simulink library "halin"  (R2021b)
settings: Solver=VariableStepAuto  StartTime=0.0  StopTime=10.0  RelTol=1e-3
undefined symbols (not defined in the file): KHAL_CAN1ABM1E2E_flg, KHAL_CAN1EPB1E2E_flg, KHAL_CAN1EPS1E2E_flg, KHAL_CAN1ESC1E2E_flg, KHAL_CAN1ESC5E2E_flg, KHAL_CAN3BMS1E2E_flg, KHAL_CAN3BMS6E2E_flg, KHAL_CAN3CCU1E2E_flg, KHAL_CAN3CCU2E2E_flg, KHAL_CAN3MCUNF1E2E_flg, KHAL_CAN3MCUNR1E2E_flg, KHAL_CAN3Shifter1E2E_flg, KHAL_CAN3Shifter2E2E_flg, KHAL_CAN6FCM2E2E_flg, KHAL_CAN6FCM4E2E_flg, TRUE
libraries: simulink x645, FVT_lib x212, hcu_lib x59
(part 4 of 23)

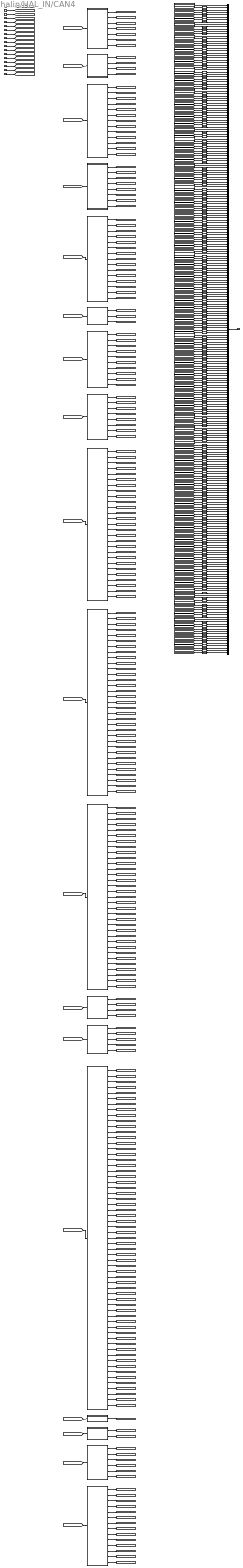
== system halin/HAL_IN/CAN4 ==
  DT_CAN4_SG_BodyZone_DR1 : Inport
  DT_CAN4_SG_BodyZone_DR2 : Inport  Port=2
  DT_CAN4_SG_BodyZone_PS1 : Inport  Port=3
  DT_CAN4_SG_BodyZone_PS2 : Inport  Port=4
  DT_CAN4_SG_DKC1 : Inport  Port=5
  DT_CAN4_SG_DKC2 : Inport  Port=6
  DT_CAN4_SG_PTG1 : Inport  Port=7
  DT_CAN4_SG_ZONE_DR1 : Inport  Port=8
  DT_CAN4_SG_ZONE_DR_VCU : Inport  Port=9
  DT_CAN4_SG_ZONE_FR1 : Inport  Port=10
  DT_CAN4_SG_ZONE_FR_VCU : Inport  Port=11
  DT_CAN4_SG_zGW_APTC1 : Inport  Port=12
  DT_CAN4_SG_zGW_CANFr1 : Inport  Port=13
  DT_CAN4_SG_zGW_LINDr1 : Inport  Port=14
  DT_CAN4_SG_zGW_LINDr2 : Inport  Port=15
  DT_CAN4_SG_zGW_LINFr1 : Inport  Port=16
  DT_CAN4_SG_zGW_LINFr2 : Inport  Port=17
  DT_CAN4_SG_zGW_SEAT1 : Inport  Port=18
  BodyZone_DR1 : Subsystem
  BodyZone_DR2 : Subsystem
  BodyZone_PS1 : Subsystem
  BodyZone_PS2 : Subsystem
  DKC1 : Subsystem
  DKC2 : Subsystem
  PTG1 : Subsystem
  UnitConverter{,1..2,9..11,16,19,26..27,44,46,51..52,55,60..62,64,66..67,69..72,95..97,99..100,102..119,121..123,138,170,173,177..179,182..183,186..187,190..191,194..195,197..231,240..242,248} (104 alike) : DataTypeConversion  OutDataTypeStr=boolean
  UnitConverter{7..8,21,24..25,56,63,65,74,76,78,80,82,84,86,88,90,92,98,101,124..127,129,131,139,141,143,145,147,149,151,153,159,161..169,180,184,188,192} (48 alike) : DataTypeConversion  OutDataTypeStr=single
  UnitConverter{3..6,12..15,17..18,22..23,28..43,45,50,53..54,57..59,68,75,77,79,81,83,85,87,89,91,93..94,120,128,130,132..137,140,142,144,146,148,150,152,154..158,160,171..172,174..176,181,185,189,193,196,232..239,244,246..247,250,252..253} (93 alike) : DataTypeConversion  OutDataTypeStr=uint8
  UnitConverter{20,73,243,245,249,251} (6 alike) : DataTypeConversion  OutDataTypeStr=uint16
  UnitConverter47 : DataTypeConversion  OutDataTypeStr=uint64
  UnitConverter48 : DataTypeConversion  OutDataTypeStr=uint64
  UnitConverter49 : DataTypeConversion  OutDataTypeStr=uint64
  VHAL_CANMsgInvalidBodyZoneDR1_flg : Subsystem  AncestorBlock=FVT_lib/hal/MsgTimeoutJudge_CAN_AUTOSAR
      mask help: MeasumentTrigerEvent
      mask Display: fprintf('MsgTimeoutJudge_CAN\nAUTOSAR');
  VHAL_CANMsgInvalidBodyZoneDR2_flg : Subsystem  AncestorBlock=FVT_lib/hal/MsgTimeoutJudge_CAN_AUTOSAR
      mask help: MeasumentTrigerEvent
      mask Display: fprintf('MsgTimeoutJudge_CAN\nAUTOSAR');
  VHAL_CANMsgInvalidBodyZonePS1_flg : Subsystem  AncestorBlock=FVT_lib/hal/MsgTimeoutJudge_CAN_AUTOSAR
      mask help: MeasumentTrigerEvent
      mask Display: fprintf('MsgTimeoutJudge_CAN\nAUTOSAR');
  VHAL_CANMsgInvalidBodyZonePS2_flg : Subsystem  AncestorBlock=FVT_lib/hal/MsgTimeoutJudge_CAN_AUTOSAR
      mask help: MeasumentTrigerEvent
      mask Display: fprintf('MsgTimeoutJudge_CAN\nAUTOSAR');
  VHAL_CANMsgInvalidDKC1_flg : Subsystem  AncestorBlock=FVT_lib/hal/MsgTimeoutJudge_CAN_AUTOSAR
      mask help: MeasumentTrigerEvent
      mask Display: fprintf('MsgTimeoutJudge_CAN\nAUTOSAR');
  VHAL_CANMsgInvalidDKC2_flg : Subsystem  AncestorBlock=FVT_lib/hal/MsgTimeoutJudge_CAN_AUTOSAR
      mask help: MeasumentTrigerEvent
      mask Display: fprintf('MsgTimeoutJudge_CAN\nAUTOSAR');
  VHAL_CANMsgInvalidPTG1_flg : Subsystem  AncestorBlock=FVT_lib/hal/MsgTimeoutJudge_CAN_AUTOSAR
      mask help: MeasumentTrigerEvent
      mask Display: fprintf('MsgTimeoutJudge_CAN\nAUTOSAR');
  VHAL_CANMsgInvalidZONEDR1_flg : Subsystem  AncestorBlock=FVT_lib/hal/MsgTimeoutJudge_CAN_AUTOSAR
      mask help: MeasumentTrigerEvent
      mask Display: fprintf('MsgTimeoutJudge_CAN\nAUTOSAR');
  VHAL_CANMsgInvalidZONEDRVCU_flg : Subsystem  AncestorBlock=FVT_lib/hal/MsgTimeoutJudge_CAN_AUTOSAR
      mask help: MeasumentTrigerEvent
      mask Display: fprintf('MsgTimeoutJudge_CAN\nAUTOSAR');
  VHAL_CANMsgInvalidZONEFR1_flg : Subsystem  AncestorBlock=FVT_lib/hal/MsgTimeoutJudge_CAN_AUTOSAR
      mask help: MeasumentTrigerEvent
      mask Display: fprintf('MsgTimeoutJudge_CAN\nAUTOSAR');
  VHAL_CANMsgInvalidZONEFRVCU_flg : Subsystem  AncestorBlock=FVT_lib/hal/MsgTimeoutJudge_CAN_AUTOSAR
      mask help: MeasumentTrigerEvent
      mask Display: fprintf('MsgTimeoutJudge_CAN\nAUTOSAR');
  VHAL_CANMsgInvalidzGWAPTC1_flg : Subsystem  AncestorBlock=FVT_lib/hal/MsgTimeoutJudge_CAN_AUTOSAR
      mask help: MeasumentTrigerEvent
      mask Display: fprintf('MsgTimeoutJudge_CAN\nAUTOSAR');
  VHAL_CANMsgInvalidzGWCANFr1_flg : Subsystem  AncestorBlock=FVT_lib/hal/MsgTimeoutJudge_CAN_AUTOSAR
      mask help: MeasumentTrigerEvent
      mask Display: fprintf('MsgTimeoutJudge_CAN\nAUTOSAR');
  VHAL_CANMsgInvalidzGWLINDr1_flg : Subsystem  AncestorBlock=FVT_lib/hal/MsgTimeoutJudge_CAN_AUTOSAR
      mask help: MeasumentTrigerEvent
      mask Display: fprintf('MsgTimeoutJudge_CAN\nAUTOSAR');
  VHAL_CANMsgInvalidzGWLINDr2_flg : Subsystem  AncestorBlock=FVT_lib/hal/MsgTimeoutJudge_CAN_AUTOSAR
      mask help: MeasumentTrigerEvent
      mask Display: fprintf('MsgTimeoutJudge_CAN\nAUTOSAR');
  VHAL_CANMsgInvalidzGWLINFr1_flg : Subsystem  AncestorBlock=FVT_lib/hal/MsgTimeoutJudge_CAN_AUTOSAR
      mask help: MeasumentTrigerEvent
      mask Display: fprintf('MsgTimeoutJudge_CAN\nAUTOSAR');
  VHAL_CANMsgInvalidzGWLINFr2_flg : Subsystem  AncestorBlock=FVT_lib/hal/MsgTimeoutJudge_CAN_AUTOSAR
      mask help: MeasumentTrigerEvent
      mask Display: fprintf('MsgTimeoutJudge_CAN\nAUTOSAR');
  VHAL_CANMsgInvalidzGWSEAT1_flg : Subsystem  AncestorBlock=FVT_lib/hal/MsgTimeoutJudge_CAN_AUTOSAR
      mask help: MeasumentTrigerEvent
      mask Display: fprintf('MsgTimeoutJudge_CAN\nAUTOSAR');
  ZONE_DR1 : Subsystem
  ZONE_DR_VCU : Subsystem
  ZONE_FR1 : Subsystem
  ZONE_FR_VCU : Subsystem
  bus_creator : BusCreator  Inputs=272
  zGW_APTC1 : Subsystem
  zGW_CANFr1 : Subsystem
  zGW_LINDr1 : Subsystem
  zGW_LINDr2 : Subsystem
  zGW_LINFr1 : Subsystem
  zGW_LINFr2 : Subsystem
  zGW_SEAT1 : Subsystem
  HAL_CAN4_outputs : Outport
  wires:
  DT_CAN4_SG_BodyZone_DR1/1 -> [DT_CAN4_SG_BodyZone_DR1]
  DT_CAN4_SG_BodyZone_DR2/1 -> [DT_CAN4_SG_BodyZone_DR2]
  DT_CAN4_SG_BodyZone_PS1/1 -> [DT_CAN4_SG_BodyZone_PS1]
  DT_CAN4_SG_BodyZone_PS2/1 -> [DT_CAN4_SG_BodyZone_PS2]
  DT_CAN4_SG_DKC1/1 -> [DT_CAN4_SG_DKC1]
  DT_CAN4_SG_DKC2/1 -> [DT_CAN4_SG_DKC2]
  DT_CAN4_SG_PTG1/1 -> [DT_CAN4_SG_PTG1]
  DT_CAN4_SG_ZONE_DR1/1 -> [DT_CAN4_SG_ZONE_DR1]
  DT_CAN4_SG_ZONE_DR_VCU/1 -> [DT_CAN4_SG_ZONE_DR_VCU]
  DT_CAN4_SG_ZONE_FR1/1 -> [DT_CAN4_SG_ZONE_FR1]
  DT_CAN4_SG_ZONE_FR_VCU/1 -> [DT_CAN4_SG_ZONE_FR_VCU]
  DT_CAN4_SG_zGW_APTC1/1 -> [DT_CAN4_SG_zGW_APTC1]
  DT_CAN4_SG_zGW_CANFr1/1 -> [DT_CAN4_SG_zGW_CANFr1]
  DT_CAN4_SG_zGW_LINDr1/1 -> [DT_CAN4_SG_zGW_LINDr1]
  DT_CAN4_SG_zGW_LINDr2/1 -> [DT_CAN4_SG_zGW_LINDr2]
  DT_CAN4_SG_zGW_LINFr1/1 -> [DT_CAN4_SG_zGW_LINFr1]
  DT_CAN4_SG_zGW_LINFr2/1 -> [DT_CAN4_SG_zGW_LINFr2]
  DT_CAN4_SG_zGW_SEAT1/1 -> [DT_CAN4_SG_zGW_SEAT1]
  [DT_CAN4_SG_BodyZone_DR1] -> BodyZone_DR1/1(DT_CAN4_SG_BodyZone_DR1)
  [DT_CAN4_SG_BodyZone_DR2] -> BodyZone_DR2/1(DT_CAN4_SG_BodyZone_DR2)
  [DT_CAN4_SG_BodyZone_PS1] -> BodyZone_PS1/1(DT_CAN4_SG_BodyZone_PS1)
  [DT_CAN4_SG_BodyZone_PS2] -> BodyZone_PS2/1(DT_CAN4_SG_BodyZone_PS2)
  [DT_CAN4_SG_DKC1] -> DKC1/1(DT_CAN4_SG_DKC1)
  [DT_CAN4_SG_DKC2] -> DKC2/1(DT_CAN4_SG_DKC2)
  [DT_CAN4_SG_PTG1] -> PTG1/1(DT_CAN4_SG_PTG1)
  [DT_CAN4_SG_ZONE_DR1] -> ZONE_DR1/1(DT_CAN4_SG_ZONE_DR1)
  [DT_CAN4_SG_ZONE_DR_VCU] -> ZONE_DR_VCU/1(DT_CAN4_SG_ZONE_DR_VCU)
  [DT_CAN4_SG_ZONE_FR1] -> ZONE_FR1/1(DT_CAN4_SG_ZONE_FR1)
  [DT_CAN4_SG_ZONE_FR_VCU] -> ZONE_FR_VCU/1(DT_CAN4_SG_ZONE_FR_VCU)
  [DT_CAN4_SG_zGW_APTC1] -> zGW_APTC1/1(DT_CAN4_SG_zGW_APTC1)
  [DT_CAN4_SG_zGW_CANFr1] -> zGW_CANFr1/1(DT_CAN4_SG_zGW_CANFr1)
  [DT_CAN4_SG_zGW_LINDr1] -> zGW_LINDr1/1(DT_CAN4_SG_zGW_LINDr1)
  [DT_CAN4_SG_zGW_LINDr2] -> zGW_LINDr2/1(DT_CAN4_SG_zGW_LINDr2)
  [DT_CAN4_SG_zGW_LINFr1] -> zGW_LINFr1/1(DT_CAN4_SG_zGW_LINFr1)
  [DT_CAN4_SG_zGW_LINFr2] -> zGW_LINFr2/1(DT_CAN4_SG_zGW_LINFr2)
  [DT_CAN4_SG_zGW_SEAT1] -> zGW_SEAT1/1(DT_CAN4_SG_zGW_SEAT1)
  bus_creator/1 -> HAL_CAN4_outputs/1
  VHAL_CANMsgInvalidBodyZoneDR1_flg/1(Out) -> bus_creator/1
  BodyZone_DR1/1(VHAL_BDDSEATAntiSta_flg) -> [VHAL_BDDSEATAntiSta_flg]
  UnitConverter/1 -> bus_creator/2  "VHAL_BDDSEATAntiSta_flg"
  [VHAL_BDDSEATAntiSta_flg] -> UnitConverter/1
  BodyZone_DR1/2(VHAL_BDDSEATEntryFunSta_flg) -> [VHAL_BDDSEATEntryFunSta_flg]
  UnitConverter1/1 -> bus_creator/3  "VHAL_BDDSEATEntryFunSta_flg"
  [VHAL_BDDSEATEntryFunSta_flg] -> UnitConverter1/1
  BodyZone_DR1/3(VHAL_BDDSEATErrorSta_flg) -> [VHAL_BDDSEATErrorSta_flg]
  UnitConverter2/1 -> bus_creator/4  "VHAL_BDDSEATErrorSta_flg"
  [VHAL_BDDSEATErrorSta_flg] -> UnitConverter2/1
  BodyZone_DR1/4(VHAL_BDDSEATMemSetSta_enum) -> [VHAL_BDDSEATMemSetSta_enum]
  UnitConverter3/1 -> bus_creator/5  "VHAL_BDDSEATMemSetSta_enum"
  [VHAL_BDDSEATMemSetSta_enum] -> UnitConverter3/1
  BodyZone_DR1/5(VHAL_BDDSEATModeSta_enum) -> [VHAL_BDDSEATModeSta_enum]
  UnitConverter4/1 -> bus_creator/6  "VHAL_BDDSEATModeSta_enum"
  [VHAL_BDDSEATModeSta_enum] -> UnitConverter4/1
  BodyZone_DR1/6(VHAL_BDDSEATVentSta_enum) -> [VHAL_BDDSEATVentSta_enum]
  UnitConverter5/1 -> bus_creator/7  "VHAL_BDDSEATVentSta_enum"
  [VHAL_BDDSEATVentSta_enum] -> UnitConverter5/1
  BodyZone_DR1/7(VHAL_BDDSEATheaterSta_enum) -> [VHAL_BDDSEATheaterSta_enum]
  UnitConverter6/1 -> bus_creator/8  "VHAL_BDDSEATheaterSta_enum"
  [VHAL_BDDSEATheaterSta_enum] -> UnitConverter6/1
  VHAL_CANMsgInvalidBodyZoneDR2_flg/1(Out) -> bus_creator/9
  BodyZone_DR2/1(VHAL_BDAPMWinFOpenedSta_pct) -> [VHAL_BDAPMWinFOpenedSta_pct]
  UnitConverter7/1 -> bus_creator/10  "VHAL_BDAPMWinFOpenedSta_pct"
  [VHAL_BDAPMWinFOpenedSta_pct] -> UnitConverter7/1
  BodyZone_DR2/2(VHAL_BDAPMWinROpenedSta_pct) -> [VHAL_BDAPMWinROpenedSta_pct]
  UnitConverter8/1 -> bus_creator/11  "VHAL_BDAPMWinROpenedSta_pct"
  [VHAL_BDAPMWinROpenedSta_pct] -> UnitConverter8/1
  BodyZone_DR2/3(VHAL_BDDoorFHandleCloseSta_flg) -> [VHAL_BDDoorFHandleCloseSta_flg]
  UnitConverter9/1 -> bus_creator/12  "VHAL_BDDoorFHandleCloseSta_flg"
  [VHAL_BDDoorFHandleCloseSta_flg] -> UnitConverter9/1
  BodyZone_DR2/4(VHAL_BDDoorRHandleCloseSta_flg) -> [VHAL_BDDoorRHandleCloseSta_flg]
  UnitConverter10/1 -> bus_creator/13  "VHAL_BDDoorRHandleCloseSta_flg"
  [VHAL_BDDoorRHandleCloseSta_flg] -> UnitConverter10/1
  VHAL_CANMsgInvalidBodyZonePS1_flg/1(Out) -> bus_creator/14
  BodyZone_PS1/1(VHAL_BPPSEATErrorSta_flg) -> [VHAL_BPPSEATErrorSta_flg]
  UnitConverter11/1 -> bus_creator/15  "VHAL_BPPSEATErrorSta_flg"
  [VHAL_BPPSEATErrorSta_flg] -> UnitConverter11/1
  BodyZone_PS1/2(VHAL_BPPSEATModeSta_enum) -> [VHAL_BPPSEATModeSta_enum]
  UnitConverter12/1 -> bus_creator/16  "VHAL_BPPSEATModeSta_enum"
  [VHAL_BPPSEATModeSta_enum] -> UnitConverter12/1
  BodyZone_PS1/3(VHAL_BPPSEATVentSta_enum) -> [VHAL_BPPSEATVentSta_enum]
  UnitConverter13/1 -> bus_creator/17  "VHAL_BPPSEATVentSta_enum"
  [VHAL_BPPSEATVentSta_enum] -> UnitConverter13/1
  BodyZone_PS1/4(VHAL_BPPSEATheaterSta_enum) -> [VHAL_BPPSEATheaterSta_enum]
  UnitConverter14/1 -> bus_creator/18  "VHAL_BPPSEATheaterSta_enum"
  [VHAL_BPPSEATheaterSta_enum] -> UnitConverter14/1
  BodyZone_PS1/5(VHAL_BPPTGActiveSta_enum) -> [VHAL_BPPTGActiveSta_enum]
  UnitConverter15/1 -> bus_creator/19  "VHAL_BPPTGActiveSta_enum"
  [VHAL_BPPTGActiveSta_enum] -> UnitConverter15/1
  BodyZone_PS1/6(VHAL_BPPTGExistSta_flg) -> [VHAL_BPPTGExistSta_flg]
  UnitConverter16/1 -> bus_creator/20  "VHAL_BPPTGExistSta_flg"
  [VHAL_BPPTGExistSta_flg] -> UnitConverter16/1
  BodyZone_PS1/7(VHAL_BPPTGInsideSW1Sta_enum) -> [VHAL_BPPTGInsideSW1Sta_enum]
  UnitConverter17/1 -> bus_creator/21  "VHAL_BPPTGInsideSW1Sta_enum"
  [VHAL_BPPTGInsideSW1Sta_enum] -> UnitConverter17/1
  BodyZone_PS1/8(VHAL_BPPTGInsideSW2Sta_enum) -> [VHAL_BPPTGInsideSW2Sta_enum]
  UnitConverter18/1 -> bus_creator/22  "VHAL_BPPTGInsideSW2Sta_enum"
  [VHAL_BPPTGInsideSW2Sta_enum] -> UnitConverter18/1
  BodyZone_PS1/9(VHAL_BPPTGIsSetHeightSta_flg) -> [VHAL_BPPTGIsSetHeightSta_flg]
  UnitConverter19/1 -> bus_creator/23  "VHAL_BPPTGIsSetHeightSta_flg"
  [VHAL_BPPTGIsSetHeightSta_flg] -> UnitConverter19/1
  BodyZone_PS1/10(VHAL_BPPTGLeftHallPosnSta_enum) -> [VHAL_BPPTGLeftHallPosnSta_enum]
  UnitConverter20/1 -> bus_creator/24  "VHAL_BPPTGLeftHallPosnSta_enum"
  [VHAL_BPPTGLeftHallPosnSta_enum] -> UnitConverter20/1
  BodyZone_PS1/11(VHAL_BPPTGOpenRatioSta_pct) -> [VHAL_BPPTGOpenRatioSta_pct]
  UnitConverter21/1 -> bus_creator/25  "VHAL_BPPTGOpenRatioSta_pct"
  [VHAL_BPPTGOpenRatioSta_pct] -> UnitConverter21/1
  BodyZone_PS1/12(VHAL_BPPTGRDILCmd_enum) -> [VHAL_BPPTGRDILCmd_enum]
  UnitConverter22/1 -> bus_creator/26  "VHAL_BPPTGRDILCmd_enum"
  [VHAL_BPPTGRDILCmd_enum] -> UnitConverter22/1
  BodyZone_PS1/13(VHAL_BPPTGSysSta_enum) -> [VHAL_BPPTGSysSta_enum]
  UnitConverter23/1 -> bus_creator/27  "VHAL_BPPTGSysSta_enum"
  [VHAL_BPPTGSysSta_enum] -> UnitConverter23/1
  VHAL_CANMsgInvalidBodyZonePS2_flg/1(Out) -> bus_creator/28
  BodyZone_PS2/1(VHAL_BPAPMWinFOpenedSta_pct) -> [VHAL_BPAPMWinFOpenedSta_pct]
  UnitConverter24/1 -> bus_creator/29  "VHAL_BPAPMWinFOpenedSta_pct"
  [VHAL_BPAPMWinFOpenedSta_pct] -> UnitConverter24/1
  BodyZone_PS2/2(VHAL_BPAPMWinROpenedSta_pct) -> [VHAL_BPAPMWinROpenedSta_pct]
  UnitConverter25/1 -> bus_creator/30  "VHAL_BPAPMWinROpenedSta_pct"
  [VHAL_BPAPMWinROpenedSta_pct] -> UnitConverter25/1
  BodyZone_PS2/3(VHAL_BPDoorFHandleCloseSta_flg) -> [VHAL_BPDoorFHandleCloseSta_flg]
  UnitConverter26/1 -> bus_creator/31  "VHAL_BPDoorFHandleCloseSta_flg"
  [VHAL_BPDoorFHandleCloseSta_flg] -> UnitConverter26/1
  BodyZone_PS2/4(VHAL_BPDoorRHandleCloseSta_flg) -> [VHAL_BPDoorRHandleCloseSta_flg]
  UnitConverter27/1 -> bus_creator/32  "VHAL_BPDoorRHandleCloseSta_flg"
  [VHAL_BPDoorRHandleCloseSta_flg] -> UnitConverter27/1
  BodyZone_PS2/5(VHAL_BPSEATLVentSta_enum) -> [VHAL_BPSEATLVentSta_enum]
  UnitConverter28/1 -> bus_creator/33  "VHAL_BPSEATLVentSta_enum"
  [VHAL_BPSEATLVentSta_enum] -> UnitConverter28/1
  BodyZone_PS2/6(VHAL_BPSEATMLVentSta_enum) -> [VHAL_BPSEATMLVentSta_enum]
  UnitConverter29/1 -> bus_creator/34  "VHAL_BPSEATMLVentSta_enum"
  [VHAL_BPSEATMLVentSta_enum] -> UnitConverter29/1
  BodyZone_PS2/7(VHAL_BPSEATMRVentSta_enum) -> [VHAL_BPSEATMRVentSta_enum]
  UnitConverter30/1 -> bus_creator/35  "VHAL_BPSEATMRVentSta_enum"
  [VHAL_BPSEATMRVentSta_enum] -> UnitConverter30/1
  BodyZone_PS2/8(VHAL_BPSEATRVentSta_enum) -> [VHAL_BPSEATRVentSta_enum]
  UnitConverter31/1 -> bus_creator/36  "VHAL_BPSEATRVentSta_enum"
  [VHAL_BPSEATRVentSta_enum] -> UnitConverter31/1
  VHAL_CANMsgInvalidDKC1_flg/1(Out) -> bus_creator/37
  DKC1/1(VHAL_DKCKeyNumSta_enum) -> [VHAL_DKCKeyNumSta_enum]
  UnitConverter32/1 -> bus_creator/38  "VHAL_DKCKeyNumSta_enum"
  [VHAL_DKCKeyNumSta_enum] -> UnitConverter32/1
  DKC1/2(VHAL_DKCKeyTypeSta_enum) -> [VHAL_DKCKeyTypeSta_enum]
  UnitConverter33/1 -> bus_creator/39  "VHAL_DKCKeyTypeSta_enum"
  [VHAL_DKCKeyTypeSta_enum] -> UnitConverter33/1
  DKC1/3(VHAL_DKCPDkeyAreaRAPSSta_enum) -> [VHAL_DKCPDkeyAreaRAPSSta_enum]
  UnitConverter34/1 -> bus_creator/40  "VHAL_DKCPDkeyAreaRAPSSta_enum"
  [VHAL_DKCPDkeyAreaRAPSSta_enum] -> UnitConverter34/1
  DKC1/4(VHAL_DKCParkingModeCmd_enum) -> [VHAL_DKCParkingModeCmd_enum]
  UnitConverter35/1 -> bus_creator/41  "VHAL_DKCParkingModeCmd_enum"
  [VHAL_DKCParkingModeCmd_enum] -> UnitConverter35/1
  DKC1/5(VHAL_DKCReVehData_enum) -> [VHAL_DKCReVehData_enum]
  UnitConverter36/1 -> bus_creator/42  "VHAL_DKCReVehData_enum"
  [VHAL_DKCReVehData_enum] -> UnitConverter36/1
  DKC1/6(VHAL_PCommandToBCM_enum) -> [VHAL_PCommandToBCM_enum]
  UnitConverter37/1 -> bus_creator/43  "VHAL_PCommandToBCM_enum"
  [VHAL_PCommandToBCM_enum] -> UnitConverter37/1
  DKC1/7(VHAL_PCommandToPTG_enum) -> [VHAL_PCommandToPTG_enum]
  UnitConverter38/1 -> bus_creator/44  "VHAL_PCommandToPTG_enum"
  [VHAL_PCommandToPTG_enum] -> UnitConverter38/1
  DKC1/8(VHAL_PDKeyAreaLockUnlock_enum) -> [VHAL_PDKeyAreaLockUnlock_enum]
  UnitConverter39/1 -> bus_creator/45  "VHAL_PDKeyAreaLockUnlock_enum"
  [VHAL_PDKeyAreaLockUnlock_enum] -> UnitConverter39/1
  DKC1/9(VHAL_PDKeyAreaPS_enum) -> [VHAL_PDKeyAreaPS_enum]
  UnitConverter40/1 -> bus_creator/46  "VHAL_PDKeyAreaPS_enum"
  [VHAL_PDKeyAreaPS_enum] -> UnitConverter40/1
  DKC1/10(VHAL_PDKeyAreaPTG_enum) -> [VHAL_PDKeyAreaPTG_enum]
  UnitConverter41/1 -> bus_creator/47  "VHAL_PDKeyAreaPTG_enum"
  [VHAL_PDKeyAreaPTG_enum] -> UnitConverter41/1
  DKC1/11(VHAL_PDKeyWelcome_enum) -> [VHAL_PDKeyWelcome_enum]
  UnitConverter42/1 -> bus_creator/48  "VHAL_PDKeyWelcome_enum"
  [VHAL_PDKeyWelcome_enum] -> UnitConverter42/1
  DKC1/12(VHAL_PDkeyShowIVI_enum) -> [VHAL_PDkeyShowIVI_enum]
  UnitConverter43/1 -> bus_creator/49  "VHAL_PDkeyShowIVI_enum"
  [VHAL_PDkeyShowIVI_enum] -> UnitConverter43/1
  DKC1/13(VHAL_PKeyMiss_flg) -> [VHAL_PKeyMiss_flg]
  UnitConverter44/1 -> bus_creator/50  "VHAL_PKeyMiss_flg"
  [VHAL_PKeyMiss_flg] -> UnitConverter44/1
  DKC1/14(VHAL_PKeyMode_enum) -> [VHAL_PKeyMode_enum]
  UnitConverter45/1 -> bus_creator/51  "VHAL_PKeyMode_enum"
  [VHAL_PKeyMode_enum] -> UnitConverter45/1
  DKC1/15(VHAL_PUIDLowPower_flg) -> [VHAL_PUIDLowPower_flg]
  UnitConverter46/1 -> bus_creator/52  "VHAL_PUIDLowPower_flg"
  [VHAL_PUIDLowPower_flg] -> UnitConverter46/1
  VHAL_CANMsgInvalidDKC2_flg/1(Out) -> bus_creator/53
  DKC2/1(VHAL_EncryptionDATA063_enum) -> [VHAL_EncryptionDATA063_enum]
  UnitConverter47/1 -> bus_creator/54  "VHAL_EncryptionDATA063_enum"
  [VHAL_EncryptionDATA063_enum] -> UnitConverter47/1
  DKC2/2(VHAL_EncryptionDATA64127_enum) -> [VHAL_EncryptionDATA64127_enum]
  UnitConverter48/1 -> bus_creator/55  "VHAL_EncryptionDATA64127_enum"
  [VHAL_EncryptionDATA64127_enum] -> UnitConverter48/1
  DKC2/3(VHAL_RandomNumberX_enum) -> [VHAL_RandomNumberX_enum]
  UnitConverter49/1 -> bus_creator/56  "VHAL_RandomNumberX_enum"
  [VHAL_RandomNumberX_enum] -> UnitConverter49/1
  VHAL_CANMsgInvalidPTG1_flg/1(Out) -> bus_creator/57
  PTG1/1(VHAL_PTGActiveSta_enum) -> [VHAL_PTGActiveSta_enum]
  UnitConverter50/1 -> bus_creator/58  "VHAL_PTGActiveSta_enum"
  [VHAL_PTGActiveSta_enum] -> UnitConverter50/1
  PTG1/2(VHAL_PTGAutoStaus_flg) -> [VHAL_PTGAutoStaus_flg]
  UnitConverter51/1 -> bus_creator/59  "VHAL_PTGAutoStaus_flg"
  [VHAL_PTGAutoStaus_flg] -> UnitConverter51/1
  PTG1/3(VHAL_PTGExist_flg) -> [VHAL_PTGExist_flg]
  UnitConverter52/1 -> bus_creator/60  "VHAL_PTGExist_flg"
  [VHAL_PTGExist_flg] -> UnitConverter52/1
  PTG1/4(VHAL_PTGHWVer_enum) -> [VHAL_PTGHWVer_enum]
  UnitConverter53/1 -> bus_creator/61  "VHAL_PTGHWVer_enum"
  [VHAL_PTGHWVer_enum] -> UnitConverter53/1
  PTG1/5(VHAL_PTGInnerSW2_enum) -> [VHAL_PTGInnerSW2_enum]
  UnitConverter54/1 -> bus_creator/62  "VHAL_PTGInnerSW2_enum"
  [VHAL_PTGInnerSW2_enum] -> UnitConverter54/1
  PTG1/6(VHAL_PTGIsSetHeight_flg) -> [VHAL_PTGIsSetHeight_flg]
  UnitConverter55/1 -> bus_creator/63  "VHAL_PTGIsSetHeight_flg"
  [VHAL_PTGIsSetHeight_flg] -> UnitConverter55/1
  PTG1/7(VHAL_PTGOpenRatio_pct) -> [VHAL_PTGOpenRatio_pct]
  UnitConverter56/1 -> bus_creator/64  "VHAL_PTGOpenRatio_pct"
  [VHAL_PTGOpenRatio_pct] -> UnitConverter56/1
  PTG1/8(VHAL_PTGRDILSta_enum) -> [VHAL_PTGRDILSta_enum]
  UnitConverter57/1 -> bus_creator/65  "VHAL_PTGRDILSta_enum"
  [VHAL_PTGRDILSta_enum] -> UnitConverter57/1
  PTG1/9(VHAL_PTGSWVer_enum) -> [VHAL_PTGSWVer_enum]
  UnitConverter58/1 -> bus_creator/66  "VHAL_PTGSWVer_enum"
  [VHAL_PTGSWVer_enum] -> UnitConverter58/1
  PTG1/10(VHAL_PTGSysSta_enum) -> [VHAL_PTGSysSta_enum]
  UnitConverter59/1 -> bus_creator/67  "VHAL_PTGSysSta_enum"
  [VHAL_PTGSysSta_enum] -> UnitConverter59/1
  VHAL_CANMsgInvalidZONEDR1_flg/1(Out) -> bus_creator/68
  ZONE_DR1/1(VHAL_DrLockSta_flg) -> [VHAL_DrLockSta_flg]
  UnitConverter60/1 -> bus_creator/69  "VHAL_DrLockSta_flg"
  [VHAL_DrLockSta_flg] -> UnitConverter60/1
  ZONE_DR1/2(VHAL_MIRRORFOLDSW_flg) -> [VHAL_MIRRORFOLDSW_flg]
  UnitConverter61/1 -> bus_creator/70  "VHAL_MIRRORFOLDSW_flg"
  [VHAL_MIRRORFOLDSW_flg] -> UnitConverter61/1
  ZONE_DR1/3(VHAL_RLTurnLPErr_flg) -> [VHAL_RLTurnLPErr_flg]
  UnitConverter62/1 -> bus_creator/71  "VHAL_RLTurnLPErr_flg"
  [VHAL_RLTurnLPErr_flg] -> UnitConverter62/1
  ZONE_DR1/4(VHAL_RLTurnLampC_mA) -> [VHAL_RLTurnLampC_mA]
  UnitConverter63/1 -> bus_creator/72  "VHAL_RLTurnLampC_mA"
  [VHAL_RLTurnLampC_mA] -> UnitConverter63/1
  ZONE_DR1/5(VHAL_RRTurnLPErr_flg) -> [VHAL_RRTurnLPErr_flg]
  UnitConverter64/1 -> bus_creator/73  "VHAL_RRTurnLPErr_flg"
  [VHAL_RRTurnLPErr_flg] -> UnitConverter64/1
  ZONE_DR1/6(VHAL_RRTurnLampC_mA) -> [VHAL_RRTurnLampC_mA]
  UnitConverter65/1 -> bus_creator/74  "VHAL_RRTurnLampC_mA"
  [VHAL_RRTurnLampC_mA] -> UnitConverter65/1
  ZONE_DR1/7(VHAL_RWiperAS_flg) -> [VHAL_RWiperAS_flg]
  UnitConverter66/1 -> bus_creator/75  "VHAL_RWiperAS_flg"
  [VHAL_RWiperAS_flg] -> UnitConverter66/1
  ZONE_DR1/8(VHAL_RWiperProtection_flg) -> [VHAL_RWiperProtection_flg]
  UnitConverter67/1 -> bus_creator/76  "VHAL_RWiperProtection_flg"
  [VHAL_RWiperProtection_flg] -> UnitConverter67/1
  VHAL_CANMsgInvalidZONEDRVCU_flg/1(Out) -> bus_creator/77
  ZONE_DR_VCU/1(VHAL_BlowerErr_enum) -> [VHAL_BlowerErr_enum]
  UnitConverter68/1 -> bus_creator/78  "VHAL_BlowerErr_enum"
  [VHAL_BlowerErr_enum] -> UnitConverter68/1
  ZONE_DR_VCU/2(VHAL_DrPMMLVOutPErrLmp_flg) -> [VHAL_DrPMMLVOutPErrLmp_flg]
  UnitConverter69/1 -> bus_creator/79  "VHAL_DrPMMLVOutPErrLmp_flg"
  [VHAL_DrPMMLVOutPErrLmp_flg] -> UnitConverter69/1
  ZONE_DR_VCU/3(VHAL_DrPMMSysErrLmp_flg) -> [VHAL_DrPMMSysErrLmp_flg]
  UnitConverter70/1 -> bus_creator/80  "VHAL_DrPMMSysErrLmp_flg"
  [VHAL_DrPMMSysErrLmp_flg] -> UnitConverter70/1
  ZONE_DR_VCU/4(VHAL_DrSCPSysErrLmp_flg) -> [VHAL_DrSCPSysErrLmp_flg]
  UnitConverter71/1 -> bus_creator/81  "VHAL_DrSCPSysErrLmp_flg"
  [VHAL_DrSCPSysErrLmp_flg] -> UnitConverter71/1
  ZONE_DR_VCU/5(VHAL_DrStdAErrSta_flg) -> [VHAL_DrStdAErrSta_flg]
  UnitConverter72/1 -> bus_creator/82  "VHAL_DrStdAErrSta_flg"
  [VHAL_DrStdAErrSta_flg] -> UnitConverter72/1
  ZONE_DR_VCU/6(VHAL_LeftHallPos_enum) -> [VHAL_LeftHallPos_enum]
  UnitConverter73/1 -> bus_creator/83  "VHAL_LeftHallPos_enum"
  [VHAL_LeftHallPos_enum] -> UnitConverter73/1
  ZONE_DR_VCU/7(VHAL_SolarL_W) -> [VHAL_SolarL_W]
  UnitConverter74/1 -> bus_creator/84  "VHAL_SolarL_W"
  [VHAL_SolarL_W] -> UnitConverter74/1
  ZONE_DR_VCU/8(VHAL_SolarLErr_enum) -> [VHAL_SolarLErr_enum]
  UnitConverter75/1 -> bus_creator/85  "VHAL_SolarLErr_enum"
  [VHAL_SolarLErr_enum] -> UnitConverter75/1
  ZONE_DR_VCU/9(VHAL_SolarR_W) -> [VHAL_SolarR_W]
  UnitConverter76/1 -> bus_creator/86  "VHAL_SolarR_W"
  [VHAL_SolarR_W] -> UnitConverter76/1
  ZONE_DR_VCU/10(VHAL_SolarRErr_enum) -> [VHAL_SolarRErr_enum]
  UnitConverter77/1 -> bus_creator/87  "VHAL_SolarRErr_enum"
  [VHAL_SolarRErr_enum] -> UnitConverter77/1
  ZONE_DR_VCU/11(VHAL_TFaceL_C) -> [VHAL_TFaceL_C]
  UnitConverter78/1 -> bus_creator/88  "VHAL_TFaceL_C"
  [VHAL_TFaceL_C] -> UnitConverter78/1
  ZONE_DR_VCU/12(VHAL_TFaceLErr_enum) -> [VHAL_TFaceLErr_enum]
  UnitConverter79/1 -> bus_creator/89  "VHAL_TFaceLErr_enum"
  [VHAL_TFaceLErr_enum] -> UnitConverter79/1
  ZONE_DR_VCU/13(VHAL_TFaceR_C) -> [VHAL_TFaceR_C]
  UnitConverter80/1 -> bus_creator/90  "VHAL_TFaceR_C"
  [VHAL_TFaceR_C] -> UnitConverter80/1
  ZONE_DR_VCU/14(VHAL_TFaceRErr_enum) -> [VHAL_TFaceRErr_enum]
  UnitConverter81/1 -> bus_creator/91  "VHAL_TFaceRErr_enum"
  [VHAL_TFaceRErr_enum] -> UnitConverter81/1
  ZONE_DR_VCU/15(VHAL_TFaceRr_C) -> [VHAL_TFaceRr_C]
  UnitConverter82/1 -> bus_creator/92  "VHAL_TFaceRr_C"
  [VHAL_TFaceRr_C] -> UnitConverter82/1
  ZONE_DR_VCU/16(VHAL_TFaceRrErr_enum) -> [VHAL_TFaceRrErr_enum]
  UnitConverter83/1 -> bus_creator/93  "VHAL_TFaceRrErr_enum"
  [VHAL_TFaceRrErr_enum] -> UnitConverter83/1
  ZONE_DR_VCU/17(VHAL_TFootL_C) -> [VHAL_TFootL_C]
  UnitConverter84/1 -> bus_creator/94  "VHAL_TFootL_C"
  [VHAL_TFootL_C] -> UnitConverter84/1
  ZONE_DR_VCU/18(VHAL_TFootLErr_enum) -> [VHAL_TFootLErr_enum]
  UnitConverter85/1 -> bus_creator/95  "VHAL_TFootLErr_enum"
  [VHAL_TFootLErr_enum] -> UnitConverter85/1
  ZONE_DR_VCU/19(VHAL_TFootR_C) -> [VHAL_TFootR_C]
  UnitConverter86/1 -> bus_creator/96  "VHAL_TFootR_C"
  [VHAL_TFootR_C] -> UnitConverter86/1
  ZONE_DR_VCU/20(VHAL_TFootRErr_enum) -> [VHAL_TFootRErr_enum]
  UnitConverter87/1 -> bus_creator/97  "VHAL_TFootRErr_enum"
  [VHAL_TFootRErr_enum] -> UnitConverter87/1
  ZONE_DR_VCU/21(VHAL_TFootRr_C) -> [VHAL_TFootRr_C]
  UnitConverter88/1 -> bus_creator/98  "VHAL_TFootRr_C"
  [VHAL_TFootRr_C] -> UnitConverter88/1
  ZONE_DR_VCU/22(VHAL_TFootRrErr_enum) -> [VHAL_TFootRrErr_enum]
  UnitConverter89/1 -> bus_creator/99  "VHAL_TFootRrErr_enum"
  [VHAL_TFootRrErr_enum] -> UnitConverter89/1
  ZONE_DR_VCU/23(VHAL_Tevap_C) -> [VHAL_Tevap_C]
  UnitConverter90/1 -> bus_creator/100  "VHAL_Tevap_C"
  [VHAL_Tevap_C] -> UnitConverter90/1
  ZONE_DR_VCU/24(VHAL_TevapErr_enum) -> [VHAL_TevapErr_enum]
  UnitConverter91/1 -> bus_creator/101  "VHAL_TevapErr_enum"
  [VHAL_TevapErr_enum] -> UnitConverter91/1
  ZONE_DR_VCU/25(VHAL_Tincar_C) -> [VHAL_Tincar_C]
  UnitConverter92/1 -> bus_creator/102  "VHAL_Tincar_C"
  [VHAL_Tincar_C] -> UnitConverter92/1
  ZONE_DR_VCU/26(VHAL_TincarErr_enum) -> [VHAL_TincarErr_enum]
  UnitConverter93/1 -> bus_creator/103  "VHAL_TincarErr_enum"
  [VHAL_TincarErr_enum] -> UnitConverter93/1
  ZONE_DR_VCU/27(VHAL_ZoneDrMalfunLevel_enum) -> [VHAL_ZoneDrMalfunLevel_enum]
  UnitConverter94/1 -> bus_creator/104  "VHAL_ZoneDrMalfunLevel_enum"
  [VHAL_ZoneDrMalfunLevel_enum] -> UnitConverter94/1
  VHAL_CANMsgInvalidZONEFR1_flg/1(Out) -> bus_creator/105
  ZONE_FR1/1(VHAL_ChargeInletLockSta_flg) -> [VHAL_ChargeInletLockSta_flg]
  UnitConverter95/1 -> bus_creator/106  "VHAL_ChargeInletLockSta_flg"
  [VHAL_ChargeInletLockSta_flg] -> UnitConverter95/1
  ZONE_FR1/2(VHAL_CompProEN_flg) -> [VHAL_CompProEN_flg]
  UnitConverter96/1 -> bus_creator/107  "VHAL_CompProEN_flg"
  [VHAL_CompProEN_flg] -> UnitConverter96/1
  ZONE_FR1/3(VHAL_FLTurnLPErr_flg) -> [VHAL_FLTurnLPErr_flg]
  UnitConverter97/1 -> bus_creator/108  "VHAL_FLTurnLPErr_flg"
  [VHAL_FLTurnLPErr_flg] -> UnitConverter97/1
  ZONE_FR1/4(VHAL_FLTurnLampC_mA) -> [VHAL_FLTurnLampC_mA]
  UnitConverter98/1 -> bus_creator/109  "VHAL_FLTurnLampC_mA"
  [VHAL_FLTurnLampC_mA] -> UnitConverter98/1
  ZONE_FR1/5(VHAL_FLTurnLightWarning_flg) -> [VHAL_FLTurnLightWarning_flg]
  UnitConverter99/1 -> bus_creator/110  "VHAL_FLTurnLightWarning_flg"
  [VHAL_FLTurnLightWarning_flg] -> UnitConverter99/1
  ZONE_FR1/6(VHAL_FRTurnLPErr_flg) -> [VHAL_FRTurnLPErr_flg]
  UnitConverter100/1 -> bus_creator/111  "VHAL_FRTurnLPErr_flg"
  [VHAL_FRTurnLPErr_flg] -> UnitConverter100/1
  ZONE_FR1/7(VHAL_FRTurnLampC_mA) -> [VHAL_FRTurnLampC_mA]
  UnitConverter101/1 -> bus_creator/112  "VHAL_FRTurnLampC_mA"
  [VHAL_FRTurnLampC_mA] -> UnitConverter101/1
  ZONE_FR1/8(VHAL_FRTurnLightWarning_flg) -> [VHAL_FRTurnLightWarning_flg]
  UnitConverter102/1 -> bus_creator/113  "VHAL_FRTurnLightWarning_flg"
  [VHAL_FRTurnLightWarning_flg] -> UnitConverter102/1
  ZONE_FR1/9(VHAL_FWiperAS_flg) -> [VHAL_FWiperAS_flg]
  UnitConverter103/1 -> bus_creator/114  "VHAL_FWiperAS_flg"
  [VHAL_FWiperAS_flg] -> UnitConverter103/1
  ZONE_FR1/10(VHAL_FWiperProtection_flg) -> [VHAL_FWiperProtection_flg]
  UnitConverter104/1 -> bus_creator/115  "VHAL_FWiperProtection_flg"
  [VHAL_FWiperProtection_flg] -> UnitConverter104/1
  ZONE_FR1/11(VHAL_LADBHibeamIndication_flg) -> [VHAL_LADBHibeamIndication_flg]
  UnitConverter105/1 -> bus_creator/116  "VHAL_LADBHibeamIndication_flg"
  [VHAL_LADBHibeamIndication_flg] -> UnitConverter105/1
  ZONE_FR1/12(VHAL_LADBOperationStatus_flg) -> [VHAL_LADBOperationStatus_flg]
  UnitConverter106/1 -> bus_creator/117  "VHAL_LADBOperationStatus_flg"
  [VHAL_LADBOperationStatus_flg] -> UnitConverter106/1
  ZONE_FR1/13(VHAL_LADBWarning_flg) -> [VHAL_LADBWarning_flg]
  UnitConverter107/1 -> bus_creator/118  "VHAL_LADBWarning_flg"
  [VHAL_LADBWarning_flg] -> UnitConverter107/1
  ZONE_FR1/14(VHAL_LAHBWarning_flg) -> [VHAL_LAHBWarning_flg]
  UnitConverter108/1 -> bus_creator/119  "VHAL_LAHBWarning_flg"
  [VHAL_LAHBWarning_flg] -> UnitConverter108/1
  ZONE_FR1/15(VHAL_LDRLWarning_flg) -> [VHAL_LDRLWarning_flg]
  UnitConverter109/1 -> bus_creator/120  "VHAL_LDRLWarning_flg"
  [VHAL_LDRLWarning_flg] -> UnitConverter109/1
  ZONE_FR1/16(VHAL_LLBWarning_flg) -> [VHAL_LLBWarning_flg]
  UnitConverter110/1 -> bus_creator/121  "VHAL_LLBWarning_flg"
  [VHAL_LLBWarning_flg] -> UnitConverter110/1
  ZONE_FR1/17(VHAL_LpositionLampWarning_flg) -> [VHAL_LpositionLampWarning_flg]
  UnitConverter111/1 -> bus_creator/122  "VHAL_LpositionLampWarning_flg"
  [VHAL_LpositionLampWarning_flg] -> UnitConverter111/1
  ZONE_FR1/18(VHAL_RADBHibeamIndication_flg) -> [VHAL_RADBHibeamIndication_flg]
  UnitConverter112/1 -> bus_creator/123  "VHAL_RADBHibeamIndication_flg"
  [VHAL_RADBHibeamIndication_flg] -> UnitConverter112/1
  ZONE_FR1/19(VHAL_RADBOperationStatus_flg) -> [VHAL_RADBOperationStatus_flg]
  UnitConverter113/1 -> bus_creator/124  "VHAL_RADBOperationStatus_flg"
  [VHAL_RADBOperationStatus_flg] -> UnitConverter113/1
  ZONE_FR1/20(VHAL_RADBWarning_flg) -> [VHAL_RADBWarning_flg]
  UnitConverter114/1 -> bus_creator/125  "VHAL_RADBWarning_flg"
  [VHAL_RADBWarning_flg] -> UnitConverter114/1
  ZONE_FR1/21(VHAL_RAHBWarning_flg) -> [VHAL_RAHBWarning_flg]
  UnitConverter115/1 -> bus_creator/126  "VHAL_RAHBWarning_flg"
  [VHAL_RAHBWarning_flg] -> UnitConverter115/1
  ZONE_FR1/22(VHAL_RDRLWarning_flg) -> [VHAL_RDRLWarning_flg]
  UnitConverter116/1 -> bus_creator/127  "VHAL_RDRLWarning_flg"
  [VHAL_RDRLWarning_flg] -> UnitConverter116/1
  ZONE_FR1/23(VHAL_RLBWarning_flg) -> [VHAL_RLBWarning_flg]
  UnitConverter117/1 -> bus_creator/128  "VHAL_RLBWarning_flg"
  [VHAL_RLBWarning_flg] -> UnitConverter117/1
  ZONE_FR1/24(VHAL_RpositionLampWarning_flg) -> [VHAL_RpositionLampWarning_flg]
  UnitConverter118/1 -> bus_creator/129  "VHAL_RpositionLampWarning_flg"
  [VHAL_RpositionLampWarning_flg] -> UnitConverter118/1
  ZONE_FR1/25(VHAL_TrailerCheck_flg) -> [VHAL_TrailerCheck_flg]
  UnitConverter119/1 -> bus_creator/130  "VHAL_TrailerCheck_flg"
  [VHAL_TrailerCheck_flg] -> UnitConverter119/1
  ZONE_FR1/26(VHAL_TrailerModeSta_enum) -> [VHAL_TrailerModeSta_enum]
  UnitConverter120/1 -> bus_creator/131  "VHAL_TrailerModeSta_enum"
  [VHAL_TrailerModeSta_enum] -> UnitConverter120/1
  ZONE_FR1/27(VHAL_ZFRBCMChargerDoorSWSta_flg) -> [VHAL_ZFRBCMChargerDoorSWSta_flg]
  UnitConverter121/1 -> bus_creator/132  "VHAL_ZFRBCMChargerDoorSWSta_flg"
  [VHAL_ZFRBCMChargerDoorSWSta_flg] -> UnitConverter121/1
  ZONE_FR1/28(VHAL_ZFRBCMHRLTurnLPNormalSta_flg) -> [VHAL_ZFRBCMHRLTurnLPNormalSta_flg]
  UnitConverter122/1 -> bus_creator/133  "VHAL_ZFRBCMHRLTurnLPNormalSta_flg"
  [VHAL_ZFRBCMHRLTurnLPNormalSta_flg] -> UnitConverter122/1
  ZONE_FR1/29(VHAL_ZFRBCMHRRTurnLPHNormalSta_flg) -> [VHAL_ZFRBCMHRRTurnLPHNormalSta_flg]
  UnitConverter123/1 -> bus_creator/134  "VHAL_ZFRBCMHRRTurnLPHNormalSta_flg"
  [VHAL_ZFRBCMHRRTurnLPHNormalSta_flg] -> UnitConverter123/1
  ZONE_FR1/30(VHAL_ZFRTHCMCLEVentActYSta_pct) -> [VHAL_ZFRTHCMCLEVentActYSta_pct]
  UnitConverter124/1 -> bus_creator/135  "VHAL_ZFRTHCMCLEVentActYSta_pct"
  [VHAL_ZFRTHCMCLEVentActYSta_pct] -> UnitConverter124/1
  ZONE_FR1/31(VHAL_ZFRTHCMCREVentActYSta_pct) -> [VHAL_ZFRTHCMCREVentActYSta_pct]
  UnitConverter125/1 -> bus_creator/136  "VHAL_ZFRTHCMCREVentActYSta_pct"
  [VHAL_ZFRTHCMCREVentActYSta_pct] -> UnitConverter125/1
  ZONE_FR1/32(VHAL_ZFRTHCMDrEVentActYSta_pct) -> [VHAL_ZFRTHCMDrEVentActYSta_pct]
  UnitConverter126/1 -> bus_creator/137  "VHAL_ZFRTHCMDrEVentActYSta_pct"
  [VHAL_ZFRTHCMDrEVentActYSta_pct] -> UnitConverter126/1
  ZONE_FR1/33(VHAL_ZFRTHCMPsEVentActYSta_pct) -> [VHAL_ZFRTHCMPsEVentActYSta_pct]
  UnitConverter127/1 -> bus_creator/138  "VHAL_ZFRTHCMPsEVentActYSta_pct"
  [VHAL_ZFRTHCMPsEVentActYSta_pct] -> UnitConverter127/1
  VHAL_CANMsgInvalidZONEFRVCU_flg/1(Out) -> bus_creator/139
  ZONE_FR_VCU/1(VHAL_AGSErr_enum) -> [VHAL_AGSErr_enum]
  UnitConverter128/1 -> bus_creator/140  "VHAL_AGSErr_enum"
  [VHAL_AGSErr_enum] -> UnitConverter128/1
  ZONE_FR_VCU/2(VHAL_BatInTemp_C) -> [VHAL_BatInTemp_C]
  UnitConverter129/1 -> bus_creator/141  "VHAL_BatInTemp_C"
  [VHAL_BatInTemp_C] -> UnitConverter129/1
  ZONE_FR_VCU/3(VHAL_BatInTempErr_enum) -> [VHAL_BatInTempErr_enum]
  UnitConverter130/1 -> bus_creator/142  "VHAL_BatInTempErr_enum"
  [VHAL_BatInTempErr_enum] -> UnitConverter130/1
  ZONE_FR_VCU/4(VHAL_BatOutTemp_C) -> [VHAL_BatOutTemp_C]
  UnitConverter131/1 -> bus_creator/143  "VHAL_BatOutTemp_C"
  [VHAL_BatOutTemp_C] -> UnitConverter131/1
  ZONE_FR_VCU/5(VHAL_COMPErr_enum) -> [VHAL_COMPErr_enum]
  UnitConverter132/1 -> bus_creator/144  "VHAL_COMPErr_enum"
  [VHAL_COMPErr_enum] -> UnitConverter132/1
  ZONE_FR_VCU/6(VHAL_EACProtectEnable_enum) -> [VHAL_EACProtectEnable_enum]
  UnitConverter133/1 -> bus_creator/145  "VHAL_EACProtectEnable_enum"
  [VHAL_EACProtectEnable_enum] -> UnitConverter133/1
  ZONE_FR_VCU/7(VHAL_EWP3Err_enum) -> [VHAL_EWP3Err_enum]
  UnitConverter134/1 -> bus_creator/146  "VHAL_EWP3Err_enum"
  [VHAL_EWP3Err_enum] -> UnitConverter134/1
  ZONE_FR_VCU/8(VHAL_EXV1Err_enum) -> [VHAL_EXV1Err_enum]
  UnitConverter135/1 -> bus_creator/147  "VHAL_EXV1Err_enum"
  [VHAL_EXV1Err_enum] -> UnitConverter135/1
  ZONE_FR_VCU/9(VHAL_EXV2Err_enum) -> [VHAL_EXV2Err_enum]
  UnitConverter136/1 -> bus_creator/148  "VHAL_EXV2Err_enum"
  [VHAL_EXV2Err_enum] -> UnitConverter136/1
  ZONE_FR_VCU/10(VHAL_FanErr_enum) -> [VHAL_FanErr_enum]
  UnitConverter137/1 -> bus_creator/149  "VHAL_FanErr_enum"
  [VHAL_FanErr_enum] -> UnitConverter137/1
  ZONE_FR_VCU/11(VHAL_FrPMMLimpHomeActReq_flg) -> [VHAL_FrPMMLimpHomeActReq_flg]
  UnitConverter138/1 -> bus_creator/150  "VHAL_FrPMMLimpHomeActReq_flg"
  [VHAL_FrPMMLimpHomeActReq_flg] -> UnitConverter138/1
  ZONE_FR_VCU/12(VHAL_MotorInTemp_C) -> [VHAL_MotorInTemp_C]
  UnitConverter139/1 -> bus_creator/151  "VHAL_MotorInTemp_C"
  [VHAL_MotorInTemp_C] -> UnitConverter139/1
  ZONE_FR_VCU/13(VHAL_MotorInTempErr_enum) -> [VHAL_MotorInTempErr_enum]
  UnitConverter140/1 -> bus_creator/152  "VHAL_MotorInTempErr_enum"
  [VHAL_MotorInTempErr_enum] -> UnitConverter140/1
  ZONE_FR_VCU/14(VHAL_MotorOutTemp_C) -> [VHAL_MotorOutTemp_C]
  UnitConverter141/1 -> bus_creator/153  "VHAL_MotorOutTemp_C"
  [VHAL_MotorOutTemp_C] -> UnitConverter141/1
  ZONE_FR_VCU/15(VHAL_MotorOutTempErr_enum) -> [VHAL_MotorOutTempErr_enum]
  UnitConverter142/1 -> bus_creator/154  "VHAL_MotorOutTempErr_enum"
  [VHAL_MotorOutTempErr_enum] -> UnitConverter142/1
  ZONE_FR_VCU/16(VHAL_PTHighP_KPa) -> [VHAL_PTHighP_KPa]
  UnitConverter143/1 -> bus_creator/155  "VHAL_PTHighP_KPa"
  [VHAL_PTHighP_KPa] -> UnitConverter143/1
  ZONE_FR_VCU/17(VHAL_PTHighPErr_enum) -> [VHAL_PTHighPErr_enum]
  UnitConverter144/1 -> bus_creator/156  "VHAL_PTHighPErr_enum"
  [VHAL_PTHighPErr_enum] -> UnitConverter144/1
  ZONE_FR_VCU/18(VHAL_PTHighTact_C) -> [VHAL_PTHighTact_C]
  UnitConverter145/1 -> bus_creator/157  "VHAL_PTHighTact_C"
  [VHAL_PTHighTact_C] -> UnitConverter145/1
  ZONE_FR_VCU/19(VHAL_PTHighTactErr_enum) -> [VHAL_PTHighTactErr_enum]
  UnitConverter146/1 -> bus_creator/158  "VHAL_PTHighTactErr_enum"
  [VHAL_PTHighTactErr_enum] -> UnitConverter146/1
  ZONE_FR_VCU/20(VHAL_PTLowP1_KPa) -> [VHAL_PTLowP1_KPa]
  UnitConverter147/1 -> bus_creator/159  "VHAL_PTLowP1_KPa"
  [VHAL_PTLowP1_KPa] -> UnitConverter147/1
  ZONE_FR_VCU/21(VHAL_PTLowP1Err_enum) -> [VHAL_PTLowP1Err_enum]
  UnitConverter148/1 -> bus_creator/160  "VHAL_PTLowP1Err_enum"
  [VHAL_PTLowP1Err_enum] -> UnitConverter148/1
  ZONE_FR_VCU/22(VHAL_PTLowP2_KPa) -> [VHAL_PTLowP2_KPa]
  UnitConverter149/1 -> bus_creator/161  "VHAL_PTLowP2_KPa"
  [VHAL_PTLowP2_KPa] -> UnitConverter149/1
  ZONE_FR_VCU/23(VHAL_PTLowP2Err_enum) -> [VHAL_PTLowP2Err_enum]
  UnitConverter150/1 -> bus_creator/162  "VHAL_PTLowP2Err_enum"
  [VHAL_PTLowP2Err_enum] -> UnitConverter150/1
  ZONE_FR_VCU/24(VHAL_PTLowT1_C) -> [VHAL_PTLowT1_C]
  UnitConverter151/1 -> bus_creator/163  "VHAL_PTLowT1_C"
  [VHAL_PTLowT1_C] -> UnitConverter151/1
  ZONE_FR_VCU/25(VHAL_PTLowT1Err_enum) -> [VHAL_PTLowT1Err_enum]
  UnitConverter152/1 -> bus_creator/164  "VHAL_PTLowT1Err_enum"
  [VHAL_PTLowT1Err_enum] -> UnitConverter152/1
  ZONE_FR_VCU/26(VHAL_PTLowT2_C) -> [VHAL_PTLowT2_C]
  UnitConverter153/1 -> bus_creator/165  "VHAL_PTLowT2_C"
  [VHAL_PTLowT2_C] -> UnitConverter153/1
  ZONE_FR_VCU/27(VHAL_PTLowT2Err_enum) -> [VHAL_PTLowT2Err_enum]
  UnitConverter154/1 -> bus_creator/166  "VHAL_PTLowT2Err_enum"
  [VHAL_PTLowT2Err_enum] -> UnitConverter154/1
  ZONE_FR_VCU/28(VHAL_SOTXVErr_enum) -> [VHAL_SOTXVErr_enum]
  UnitConverter155/1 -> bus_creator/167  "VHAL_SOTXVErr_enum"
  [VHAL_SOTXVErr_enum] -> UnitConverter155/1
  ZONE_FR_VCU/29(VHAL_SOV1Err_enum) -> [VHAL_SOV1Err_enum]
  UnitConverter156/1 -> bus_creator/168  "VHAL_SOV1Err_enum"
  [VHAL_SOV1Err_enum] -> UnitConverter156/1
  ZONE_FR_VCU/30(VHAL_SOV2Err_enum) -> [VHAL_SOV2Err_enum]
  UnitConverter157/1 -> bus_creator/169  "VHAL_SOV2Err_enum"
  [VHAL_SOV2Err_enum] -> UnitConverter157/1
  ZONE_FR_VCU/31(VHAL_SOV3Err_enum) -> [VHAL_SOV3Err_enum]
  UnitConverter158/1 -> bus_creator/170  "VHAL_SOV3Err_enum"
  [VHAL_SOV3Err_enum] -> UnitConverter158/1
  ZONE_FR_VCU/32(VHAL_Tamb_C) -> [VHAL_Tamb_C]
  UnitConverter159/1 -> bus_creator/171  "VHAL_Tamb_C"
  [VHAL_Tamb_C] -> UnitConverter159/1
  ZONE_FR_VCU/33(VHAL_TambErr_enum) -> [VHAL_TambErr_enum]
  UnitConverter160/1 -> bus_creator/172  "VHAL_TambErr_enum"
  [VHAL_TambErr_enum] -> UnitConverter160/1
  VHAL_CANMsgInvalidzGWAPTC1_flg/1(Out) -> bus_creator/173
  zGW_APTC1/1(VHAL_FrntPTCLeActHeatPwr_W) -> [VHAL_FrntPTCLeActHeatPwr_W]
  UnitConverter161/1 -> bus_creator/174  "VHAL_FrntPTCLeActHeatPwr_W"
  [VHAL_FrntPTCLeActHeatPwr_W] -> UnitConverter161/1
  zGW_APTC1/2(VHAL_FrntPTCRearLeActHeatPwr_W) -> [VHAL_FrntPTCRearLeActHeatPwr_W]
  UnitConverter162/1 -> bus_creator/175  "VHAL_FrntPTCRearLeActHeatPwr_W"
  [VHAL_FrntPTCRearLeActHeatPwr_W] -> UnitConverter162/1
  zGW_APTC1/3(VHAL_FrntPTCRearRiActHeatPwr_W) -> [VHAL_FrntPTCRearRiActHeatPwr_W]
  UnitConverter163/1 -> bus_creator/176  "VHAL_FrntPTCRearRiActHeatPwr_W"
  [VHAL_FrntPTCRearRiActHeatPwr_W] -> UnitConverter163/1
  zGW_APTC1/4(VHAL_FrntPTCRiActHeatPwr_W) -> [VHAL_FrntPTCRiActHeatPwr_W]
  UnitConverter164/1 -> bus_creator/177  "VHAL_FrntPTCRiActHeatPwr_W"
  [VHAL_FrntPTCRiActHeatPwr_W] -> UnitConverter164/1
  VHAL_CANMsgInvalidzGWCANFr1_flg/1(Out) -> bus_creator/178
  zGW_CANFr1/1(VHAL_COMPActualPwr_W) -> [VHAL_COMPActualPwr_W]
  UnitConverter165/1 -> bus_creator/179  "VHAL_COMPActualPwr_W"
  [VHAL_COMPActualPwr_W] -> UnitConverter165/1
  zGW_CANFr1/2(VHAL_COMPConCur_A) -> [VHAL_COMPConCur_A]
  UnitConverter166/1 -> bus_creator/180  "VHAL_COMPConCur_A"
  [VHAL_COMPConCur_A] -> UnitConverter166/1
  zGW_CANFr1/3(VHAL_COMPConVolt_V) -> [VHAL_COMPConVolt_V]
  UnitConverter167/1 -> bus_creator/181  "VHAL_COMPConVolt_V"
  [VHAL_COMPConVolt_V] -> UnitConverter167/1
  zGW_CANFr1/4(VHAL_COMPStatorSpd_rpm) -> [VHAL_COMPStatorSpd_rpm]
  UnitConverter168/1 -> bus_creator/182  "VHAL_COMPStatorSpd_rpm"
  [VHAL_COMPStatorSpd_rpm] -> UnitConverter168/1
  zGW_CANFr1/5(VHAL_PTC1PowerConsumption_kW) -> [VHAL_PTC1PowerConsumption_kW]
  UnitConverter169/1 -> bus_creator/183  "VHAL_PTC1PowerConsumption_kW"
  [VHAL_PTC1PowerConsumption_kW] -> UnitConverter169/1
  VHAL_CANMsgInvalidzGWLINDr1_flg/1(Out) -> bus_creator/184
  zGW_LINDr1/1(VHAL_CSWDimSw_flg) -> [VHAL_CSWDimSw_flg]
  UnitConverter170/1 -> bus_creator/185  "VHAL_CSWDimSw_flg"
  [VHAL_CSWDimSw_flg] -> UnitConverter170/1
  zGW_LINDr1/2(VHAL_CSWFWasSwSta_enum) -> [VHAL_CSWFWasSwSta_enum]
  UnitConverter171/1 -> bus_creator/186  "VHAL_CSWFWasSwSta_enum"
  [VHAL_CSWFWasSwSta_enum] -> UnitConverter171/1
  zGW_LINDr1/3(VHAL_CSWFWipSwSta_enum) -> [VHAL_CSWFWipSwSta_enum]
  UnitConverter172/1 -> bus_creator/187  "VHAL_CSWFWipSwSta_enum"
  [VHAL_CSWFWipSwSta_enum] -> UnitConverter172/1
  zGW_LINDr1/4(VHAL_CSWPassSWSta_flg) -> [VHAL_CSWPassSWSta_flg]
  UnitConverter173/1 -> bus_creator/188  "VHAL_CSWPassSWSta_flg"
  [VHAL_CSWPassSWSta_flg] -> UnitConverter173/1
  zGW_LINDr1/5(VHAL_CSWRWasSWSta_enum) -> [VHAL_CSWRWasSWSta_enum]
  UnitConverter174/1 -> bus_creator/189  "VHAL_CSWRWasSWSta_enum"
  [VHAL_CSWRWasSWSta_enum] -> UnitConverter174/1
  zGW_LINDr1/6(VHAL_CSWRWipIntSwSta_enum) -> [VHAL_CSWRWipIntSwSta_enum]
  UnitConverter175/1 -> bus_creator/190  "VHAL_CSWRWipIntSwSta_enum"
  [VHAL_CSWRWipIntSwSta_enum] -> UnitConverter175/1
  zGW_LINDr1/7(VHAL_CSWTurnSwSta_enum) -> [VHAL_CSWTurnSwSta_enum]
  UnitConverter176/1 -> bus_creator/191  "VHAL_CSWTurnSwSta_enum"
  [VHAL_CSWTurnSwSta_enum] -> UnitConverter176/1
  zGW_LINDr1/8(VHAL_FAPWL01LINResponseError_flg) -> [VHAL_FAPWL01LINResponseError_flg]
  UnitConverter177/1 -> bus_creator/192  "VHAL_FAPWL01LINResponseError_flg"
  [VHAL_FAPWL01LINResponseError_flg] -> UnitConverter177/1
  zGW_LINDr1/9(VHAL_LDrvMotorRelayError_flg) -> [VHAL_LDrvMotorRelayError_flg]
  UnitConverter178/1 -> bus_creator/193  "VHAL_LDrvMotorRelayError_flg"
  [VHAL_LDrvMotorRelayError_flg] -> UnitConverter178/1
  zGW_LINDr1/10(VHAL_LDrvMotorRippleError_flg) -> [VHAL_LDrvMotorRippleError_flg]
  UnitConverter179/1 -> bus_creator/194  "VHAL_LDrvMotorRippleError_flg"
  [VHAL_LDrvMotorRippleError_flg] -> UnitConverter179/1
  zGW_LINDr1/11(VHAL_LDrvValWdwOpened_pct) -> [VHAL_LDrvValWdwOpened_pct]
  UnitConverter180/1 -> bus_creator/195  "VHAL_LDrvValWdwOpened_pct"
  [VHAL_LDrvValWdwOpened_pct] -> UnitConverter180/1
  zGW_LINDr1/12(VHAL_LDrvWdwPositionSts_enum) -> [VHAL_LDrvWdwPositionSts_enum]
  UnitConverter181/1 -> bus_creator/196  "VHAL_LDrvWdwPositionSts_enum"
  [VHAL_LDrvWdwPositionSts_enum] -> UnitConverter181/1
  zGW_LINDr1/13(VHAL_LPasMotorRelayError_flg) -> [VHAL_LPasMotorRelayError_flg]
  UnitConverter182/1 -> bus_creator/197  "VHAL_LPasMotorRelayError_flg"
  [VHAL_LPasMotorRelayError_flg] -> UnitConverter182/1
  zGW_LINDr1/14(VHAL_LPasMotorRippleError_flg) -> [VHAL_LPasMotorRippleError_flg]
  UnitConverter183/1 -> bus_creator/198  "VHAL_LPasMotorRippleError_flg"
  [VHAL_LPasMotorRippleError_flg] -> UnitConverter183/1
  zGW_LINDr1/15(VHAL_LPasValWdwOpened_pct) -> [VHAL_LPasValWdwOpened_pct]
  UnitConverter184/1 -> bus_creator/199  "VHAL_LPasValWdwOpened_pct"
  [VHAL_LPasValWdwOpened_pct] -> UnitConverter184/1
  zGW_LINDr1/16(VHAL_LPasWdwPositionSts_enum) -> [VHAL_LPasWdwPositionSts_enum]
  UnitConverter185/1 -> bus_creator/200  "VHAL_LPasWdwPositionSts_enum"
  [VHAL_LPasWdwPositionSts_enum] -> UnitConverter185/1
  zGW_LINDr1/17(VHAL_LRLDMotorRelayError_flg) -> [VHAL_LRLDMotorRelayError_flg]
  UnitConverter186/1 -> bus_creator/201  "VHAL_LRLDMotorRelayError_flg"
  [VHAL_LRLDMotorRelayError_flg] -> UnitConverter186/1
  zGW_LINDr1/18(VHAL_LRLDMotorRippleError_flg) -> [VHAL_LRLDMotorRippleError_flg]
  UnitConverter187/1 -> bus_creator/202  "VHAL_LRLDMotorRippleError_flg"
  [VHAL_LRLDMotorRippleError_flg] -> UnitConverter187/1
  zGW_LINDr1/19(VHAL_LRLDValWdwOpened_pct) -> [VHAL_LRLDValWdwOpened_pct]
  UnitConverter188/1 -> bus_creator/203  "VHAL_LRLDValWdwOpened_pct"
  [VHAL_LRLDValWdwOpened_pct] -> UnitConverter188/1
  zGW_LINDr1/20(VHAL_LRLDWdwPositionSts_enum) -> [VHAL_LRLDWdwPositionSts_enum]
  UnitConverter189/1 -> bus_creator/204  "VHAL_LRLDWdwPositionSts_enum"
  [VHAL_LRLDWdwPositionSts_enum] -> UnitConverter189/1
  zGW_LINDr1/21(VHAL_LRRDMotorRelayError_flg) -> [VHAL_LRRDMotorRelayError_flg]
  UnitConverter190/1 -> bus_creator/205  "VHAL_LRRDMotorRelayError_flg"
  [VHAL_LRRDMotorRelayError_flg] -> UnitConverter190/1
  zGW_LINDr1/22(VHAL_LRRDMotorRippleError_flg) -> [VHAL_LRRDMotorRippleError_flg]
  UnitConverter191/1 -> bus_creator/206  "VHAL_LRRDMotorRippleError_flg"
  [VHAL_LRRDMotorRippleError_flg] -> UnitConverter191/1
  zGW_LINDr1/23(VHAL_LRRDValWdwOpened_pct) -> [VHAL_LRRDValWdwOpened_pct]
  UnitConverter192/1 -> bus_creator/207  "VHAL_LRRDValWdwOpened_pct"
  [VHAL_LRRDValWdwOpened_pct] -> UnitConverter192/1
  zGW_LINDr1/24(VHAL_LRRDWdwPositionSts_enum) -> [VHAL_LRRDWdwPositionSts_enum]
  UnitConverter193/1 -> bus_creator/208  "VHAL_LRRDWdwPositionSts_enum"
  [VHAL_LRRDWdwPositionSts_enum] -> UnitConverter193/1
  zGW_LINDr1/25(VHAL_RAPWL01LINResponseError_flg) -> [VHAL_RAPWL01LINResponseError_flg]
  UnitConverter194/1 -> bus_creator/209  "VHAL_RAPWL01LINResponseError_flg"
  [VHAL_RAPWL01LINResponseError_flg] -> UnitConverter194/1
  zGW_LINDr1/26(VHAL_RLSLampSta_flg) -> [VHAL_RLSLampSta_flg]
  UnitConverter195/1 -> bus_creator/210  "VHAL_RLSLampSta_flg"
  [VHAL_RLSLampSta_flg] -> UnitConverter195/1
  zGW_LINDr1/27(VHAL_RLSRainSnrWiperCmd_enum) -> [VHAL_RLSRainSnrWiperCmd_enum]
  UnitConverter196/1 -> bus_creator/211  "VHAL_RLSRainSnrWiperCmd_enum"
  [VHAL_RLSRainSnrWiperCmd_enum] -> UnitConverter196/1
  zGW_LINDr1/28(VHAL_SWC2LADASSta_flg) -> [VHAL_SWC2LADASSta_flg]
  UnitConverter197/1 -> bus_creator/212  "VHAL_SWC2LADASSta_flg"
  [VHAL_SWC2LADASSta_flg] -> UnitConverter197/1
  zGW_LINDr1/29(VHAL_SWC2LDriveModeSta_flg) -> [VHAL_SWC2LDriveModeSta_flg]
  UnitConverter198/1 -> bus_creator/213  "VHAL_SWC2LDriveModeSta_flg"
  [VHAL_SWC2LDriveModeSta_flg] -> UnitConverter198/1
  zGW_LINDr1/30(VHAL_SWC2LHomeSta_flg) -> [VHAL_SWC2LHomeSta_flg]
  UnitConverter199/1 -> bus_creator/214  "VHAL_SWC2LHomeSta_flg"
  [VHAL_SWC2LHomeSta_flg] -> UnitConverter199/1
  zGW_LINDr1/31(VHAL_SWC2LLeftSta_flg) -> [VHAL_SWC2LLeftSta_flg]
  UnitConverter200/1 -> bus_creator/215  "VHAL_SWC2LLeftSta_flg"
  [VHAL_SWC2LLeftSta_flg] -> UnitConverter200/1
  zGW_LINDr1/32(VHAL_SWC2LRegenUpSta_flg) -> [VHAL_SWC2LRegenUpSta_flg]
  UnitConverter201/1 -> bus_creator/216  "VHAL_SWC2LRegenUpSta_flg"
  [VHAL_SWC2LRegenUpSta_flg] -> UnitConverter201/1
  zGW_LINDr1/33(VHAL_SWC2LRightSta_flg) -> [VHAL_SWC2LRightSta_flg]
  UnitConverter202/1 -> bus_creator/217  "VHAL_SWC2LRightSta_flg"
  [VHAL_SWC2LRightSta_flg] -> UnitConverter202/1
  zGW_LINDr1/34(VHAL_SWC2LScrollDownSta_flg) -> [VHAL_SWC2LScrollDownSta_flg]
  UnitConverter203/1 -> bus_creator/218  "VHAL_SWC2LScrollDownSta_flg"
  [VHAL_SWC2LScrollDownSta_flg] -> UnitConverter203/1
  zGW_LINDr1/35(VHAL_SWC2LScrollPressSta_flg) -> [VHAL_SWC2LScrollPressSta_flg]
  UnitConverter204/1 -> bus_creator/219  "VHAL_SWC2LScrollPressSta_flg"
  [VHAL_SWC2LScrollPressSta_flg] -> UnitConverter204/1
  zGW_LINDr1/36(VHAL_SWC2LScrollUpSta_flg) -> [VHAL_SWC2LScrollUpSta_flg]
  UnitConverter205/1 -> bus_creator/220  "VHAL_SWC2LScrollUpSta_flg"
  [VHAL_SWC2LScrollUpSta_flg] -> UnitConverter205/1
  zGW_LINDr1/37(VHAL_SWC2RCustomizeSta_flg) -> [VHAL_SWC2RCustomizeSta_flg]
  UnitConverter206/1 -> bus_creator/221  "VHAL_SWC2RCustomizeSta_flg"
  [VHAL_SWC2RCustomizeSta_flg] -> UnitConverter206/1
  zGW_LINDr1/38(VHAL_SWC2RLeftSta_flg) -> [VHAL_SWC2RLeftSta_flg]
  UnitConverter207/1 -> bus_creator/222  "VHAL_SWC2RLeftSta_flg"
  [VHAL_SWC2RLeftSta_flg] -> UnitConverter207/1
  zGW_LINDr1/39(VHAL_SWC2RPageSwitchSta_flg) -> [VHAL_SWC2RPageSwitchSta_flg]
  UnitConverter208/1 -> bus_creator/223  "VHAL_SWC2RPageSwitchSta_flg"
  [VHAL_SWC2RPageSwitchSta_flg] -> UnitConverter208/1
  zGW_LINDr1/40(VHAL_SWC2RRegenDownSta_flg) -> [VHAL_SWC2RRegenDownSta_flg]
  UnitConverter209/1 -> bus_creator/224  "VHAL_SWC2RRegenDownSta_flg"
  [VHAL_SWC2RRegenDownSta_flg] -> UnitConverter209/1
  zGW_LINDr1/41(VHAL_SWC2RRightSta_flg) -> [VHAL_SWC2RRightSta_flg]
  UnitConverter210/1 -> bus_creator/225  "VHAL_SWC2RRightSta_flg"
  [VHAL_SWC2RRightSta_flg] -> UnitConverter210/1
  zGW_LINDr1/42(VHAL_SWC2RScrollDownSta_flg) -> [VHAL_SWC2RScrollDownSta_flg]
  UnitConverter211/1 -> bus_creator/226  "VHAL_SWC2RScrollDownSta_flg"
  [VHAL_SWC2RScrollDownSta_flg] -> UnitConverter211/1
  zGW_LINDr1/43(VHAL_SWC2RScrollPressSta_flg) -> [VHAL_SWC2RScrollPressSta_flg]
  UnitConverter212/1 -> bus_creator/227  "VHAL_SWC2RScrollPressSta_flg"
  [VHAL_SWC2RScrollPressSta_flg] -> UnitConverter212/1
  zGW_LINDr1/44(VHAL_SWC2RScrollUpSta_flg) -> [VHAL_SWC2RScrollUpSta_flg]
  UnitConverter213/1 -> bus_creator/228  "VHAL_SWC2RScrollUpSta_flg"
  [VHAL_SWC2RScrollUpSta_flg] -> UnitConverter213/1
  zGW_LINDr1/45(VHAL_SWC2RVRSta_flg) -> [VHAL_SWC2RVRSta_flg]
  UnitConverter214/1 -> bus_creator/229  "VHAL_SWC2RVRSta_flg"
  [VHAL_SWC2RVRSta_flg] -> UnitConverter214/1
  zGW_LINDr1/46(VHAL_SWCACCSta_flg) -> [VHAL_SWCACCSta_flg]
  UnitConverter215/1 -> bus_creator/230  "VHAL_SWCACCSta_flg"
  [VHAL_SWCACCSta_flg] -> UnitConverter215/1
  zGW_LINDr1/47(VHAL_SWCCANCELSta_flg) -> [VHAL_SWCCANCELSta_flg]
  UnitConverter216/1 -> bus_creator/231  "VHAL_SWCCANCELSta_flg"
  [VHAL_SWCCANCELSta_flg] -> UnitConverter216/1
  zGW_LINDr1/48(VHAL_SWCDistanceSta_flg) -> [VHAL_SWCDistanceSta_flg]
  UnitConverter217/1 -> bus_creator/232  "VHAL_SWCDistanceSta_flg"
  [VHAL_SWCDistanceSta_flg] -> UnitConverter217/1
  zGW_LINDr1/49(VHAL_SWCDownSta_flg) -> [VHAL_SWCDownSta_flg]
  UnitConverter218/1 -> bus_creator/233  "VHAL_SWCDownSta_flg"
  [VHAL_SWCDownSta_flg] -> UnitConverter218/1
  zGW_LINDr1/50(VHAL_SWCLKASta_flg) -> [VHAL_SWCLKASta_flg]
  UnitConverter219/1 -> bus_creator/234  "VHAL_SWCLKASta_flg"
  [VHAL_SWCLKASta_flg] -> UnitConverter219/1
  zGW_LINDr1/51(VHAL_SWCLeftSta_flg) -> [VHAL_SWCLeftSta_flg]
  UnitConverter220/1 -> bus_creator/235  "VHAL_SWCLeftSta_flg"
  [VHAL_SWCLeftSta_flg] -> UnitConverter220/1
  zGW_LINDr1/52(VHAL_SWCRegenDown_flg) -> [VHAL_SWCRegenDown_flg]
  UnitConverter221/1 -> bus_creator/236  "VHAL_SWCRegenDown_flg"
  [VHAL_SWCRegenDown_flg] -> UnitConverter221/1
  zGW_LINDr1/53(VHAL_SWCRegenUp_flg) -> [VHAL_SWCRegenUp_flg]
  UnitConverter222/1 -> bus_creator/237  "VHAL_SWCRegenUp_flg"
  [VHAL_SWCRegenUp_flg] -> UnitConverter222/1
  zGW_LINDr1/54(VHAL_SWCResUpSta_flg) -> [VHAL_SWCResUpSta_flg]
  UnitConverter223/1 -> bus_creator/238  "VHAL_SWCResUpSta_flg"
  [VHAL_SWCResUpSta_flg] -> UnitConverter223/1
  zGW_LINDr1/55(VHAL_SWCRightSta_flg) -> [VHAL_SWCRightSta_flg]
  UnitConverter224/1 -> bus_creator/239  "VHAL_SWCRightSta_flg"
  [VHAL_SWCRightSta_flg] -> UnitConverter224/1
  zGW_LINDr1/56(VHAL_SWCSetdownSta_flg) -> [VHAL_SWCSetdownSta_flg]
  UnitConverter225/1 -> bus_creator/240  "VHAL_SWCSetdownSta_flg"
  [VHAL_SWCSetdownSta_flg] -> UnitConverter225/1
  zGW_LINDr1/57(VHAL_SWCTripSta_flg) -> [VHAL_SWCTripSta_flg]
  UnitConverter226/1 -> bus_creator/241  "VHAL_SWCTripSta_flg"
  [VHAL_SWCTripSta_flg] -> UnitConverter226/1
  zGW_LINDr1/58(VHAL_SWCUndefinedSta_flg) -> [VHAL_SWCUndefinedSta_flg]
  UnitConverter227/1 -> bus_creator/242  "VHAL_SWCUndefinedSta_flg"
  [VHAL_SWCUndefinedSta_flg] -> UnitConverter227/1
  zGW_LINDr1/59(VHAL_SWCUpSta_flg) -> [VHAL_SWCUpSta_flg]
  UnitConverter228/1 -> bus_creator/243  "VHAL_SWCUpSta_flg"
  [VHAL_SWCUpSta_flg] -> UnitConverter228/1
  zGW_LINDr1/60(VHAL_SWCVRSta_flg) -> [VHAL_SWCVRSta_flg]
  UnitConverter229/1 -> bus_creator/244  "VHAL_SWCVRSta_flg"
  [VHAL_SWCVRSta_flg] -> UnitConverter229/1
  zGW_LINDr1/61(VHAL_SWCmodeSta_flg) -> [VHAL_SWCmodeSta_flg]
  UnitConverter230/1 -> bus_creator/245  "VHAL_SWCmodeSta_flg"
  [VHAL_SWCmodeSta_flg] -> UnitConverter230/1
  VHAL_CANMsgInvalidzGWLINDr2_flg/1(Out) -> bus_creator/246
  zGW_LINDr2/1(VHAL_ACT1ResponseError_flg) -> [VHAL_ACT1ResponseError_flg]
  UnitConverter231/1 -> bus_creator/247  "VHAL_ACT1ResponseError_flg"
  [VHAL_ACT1ResponseError_flg] -> UnitConverter231/1
  VHAL_CANMsgInvalidzGWLINFr1_flg/1(Out) -> bus_creator/248
  zGW_LINFr1/1(VHAL_AGSActualPosition_enum) -> [VHAL_AGSActualPosition_enum]
  UnitConverter232/1 -> bus_creator/249  "VHAL_AGSActualPosition_enum"
  [VHAL_AGSActualPosition_enum] -> UnitConverter232/1
  zGW_LINFr1/2(VHAL_FGSIntenRspSta_enum) -> [VHAL_FGSIntenRspSta_enum]
  UnitConverter233/1 -> bus_creator/250  "VHAL_FGSIntenRspSta_enum"
  [VHAL_FGSIntenRspSta_enum] -> UnitConverter233/1
  VHAL_CANMsgInvalidzGWLINFr2_flg/1(Out) -> bus_creator/251
  zGW_LINFr2/1(VHAL_EWP1BlockError_enum) -> [VHAL_EWP1BlockError_enum]
  UnitConverter234/1 -> bus_creator/252  "VHAL_EWP1BlockError_enum"
  [VHAL_EWP1BlockError_enum] -> UnitConverter234/1
  zGW_LINFr2/2(VHAL_EWP1OverCurrError_enum) -> [VHAL_EWP1OverCurrError_enum]
  UnitConverter235/1 -> bus_creator/253  "VHAL_EWP1OverCurrError_enum"
  [VHAL_EWP1OverCurrError_enum] -> UnitConverter235/1
  zGW_LINFr2/3(VHAL_EWP2BlockError_enum) -> [VHAL_EWP2BlockError_enum]
  UnitConverter236/1 -> bus_creator/254  "VHAL_EWP2BlockError_enum"
  [VHAL_EWP2BlockError_enum] -> UnitConverter236/1
  zGW_LINFr2/4(VHAL_EWP2OverCurrError_enum) -> [VHAL_EWP2OverCurrError_enum]
  UnitConverter237/1 -> bus_creator/255  "VHAL_EWP2OverCurrError_enum"
  [VHAL_EWP2OverCurrError_enum] -> UnitConverter237/1
  zGW_LINFr2/5(VHAL_EWP3BlockError_enum) -> [VHAL_EWP3BlockError_enum]
  UnitConverter238/1 -> bus_creator/256  "VHAL_EWP3BlockError_enum"
  [VHAL_EWP3BlockError_enum] -> UnitConverter238/1
  zGW_LINFr2/6(VHAL_EWP3OverCurrError_enum) -> [VHAL_EWP3OverCurrError_enum]
  UnitConverter239/1 -> bus_creator/257  "VHAL_EWP3OverCurrError_enum"
  [VHAL_EWP3OverCurrError_enum] -> UnitConverter239/1
  VHAL_CANMsgInvalidzGWSEAT1_flg/1(Out) -> bus_creator/258
  zGW_SEAT1/1(VHAL_DSEATAntiSta_flg) -> [VHAL_DSEATAntiSta_flg]
  UnitConverter240/1 -> bus_creator/259  "VHAL_DSEATAntiSta_flg"
  [VHAL_DSEATAntiSta_flg] -> UnitConverter240/1
  zGW_SEAT1/2(VHAL_DSEATEntryFunSta_flg) -> [VHAL_DSEATEntryFunSta_flg]
  UnitConverter241/1 -> bus_creator/260  "VHAL_DSEATEntryFunSta_flg"
  [VHAL_DSEATEntryFunSta_flg] -> UnitConverter241/1
  zGW_SEAT1/3(VHAL_DSEATErrorSta_flg) -> [VHAL_DSEATErrorSta_flg]
  UnitConverter242/1 -> bus_creator/261  "VHAL_DSEATErrorSta_flg"
  [VHAL_DSEATErrorSta_flg] -> UnitConverter242/1
  zGW_SEAT1/4(VHAL_DSEATHWVer_enum) -> [VHAL_DSEATHWVer_enum]
  UnitConverter243/1 -> bus_creator/262  "VHAL_DSEATHWVer_enum"
  [VHAL_DSEATHWVer_enum] -> UnitConverter243/1
  zGW_SEAT1/5(VHAL_DSEATMode_enum) -> [VHAL_DSEATMode_enum]
  UnitConverter244/1 -> bus_creator/263  "VHAL_DSEATMode_enum"
  [VHAL_DSEATMode_enum] -> UnitConverter244/1
  zGW_SEAT1/6(VHAL_DSEATSWVer_enum) -> [VHAL_DSEATSWVer_enum]
  UnitConverter245/1 -> bus_creator/264  "VHAL_DSEATSWVer_enum"
  [VHAL_DSEATSWVer_enum] -> UnitConverter245/1
  zGW_SEAT1/7(VHAL_DSEATVentSta_enum) -> [VHAL_DSEATVentSta_enum]
  UnitConverter246/1 -> bus_creator/265  "VHAL_DSEATVentSta_enum"
  [VHAL_DSEATVentSta_enum] -> UnitConverter246/1
  zGW_SEAT1/8(VHAL_DSEATheatersta_enum) -> [VHAL_DSEATheatersta_enum]
  UnitConverter247/1 -> bus_creator/266  "VHAL_DSEATheatersta_enum"
  [VHAL_DSEATheatersta_enum] -> UnitConverter247/1
  zGW_SEAT1/9(VHAL_PSEATErrorSta_flg) -> [VHAL_PSEATErrorSta_flg]
  UnitConverter248/1 -> bus_creator/267  "VHAL_PSEATErrorSta_flg"
  [VHAL_PSEATErrorSta_flg] -> UnitConverter248/1
  zGW_SEAT1/10(VHAL_PSEATHWVer_enum) -> [VHAL_PSEATHWVer_enum]
  UnitConverter249/1 -> bus_creator/268  "VHAL_PSEATHWVer_enum"
  [VHAL_PSEATHWVer_enum] -> UnitConverter249/1
  zGW_SEAT1/11(VHAL_PSEATMode_enum) -> [VHAL_PSEATMode_enum]
  UnitConverter250/1 -> bus_creator/269  "VHAL_PSEATMode_enum"
  [VHAL_PSEATMode_enum] -> UnitConverter250/1
  zGW_SEAT1/12(VHAL_PSEATSWVer_enum) -> [VHAL_PSEATSWVer_enum]
  UnitConverter251/1 -> bus_creator/270  "VHAL_PSEATSWVer_enum"
  [VHAL_PSEATSWVer_enum] -> UnitConverter251/1
  zGW_SEAT1/13(VHAL_PSEATVentSta_enum) -> [VHAL_PSEATVentSta_enum]
  UnitConverter252/1 -> bus_creator/271  "VHAL_PSEATVentSta_enum"
  [VHAL_PSEATVentSta_enum] -> UnitConverter252/1
  zGW_SEAT1/14(VHAL_PSEATheatersta_enum) -> [VHAL_PSEATheatersta_enum]
  UnitConverter253/1 -> bus_creator/272  "VHAL_PSEATheatersta_enum"
  [VHAL_PSEATheatersta_enum] -> UnitConverter253/1
